simulink model "control_modos_deslizantes"  (R2016a)
settings: Solver=VariableStepAuto  StartTime=0.0  StopTime=20  RelTol=1e-3
undefined symbols (not defined in the file or in its folder): A, a0, a1, B, C, eta
settings Model: Creator=Daniel  LastModifiedBy=Daniel

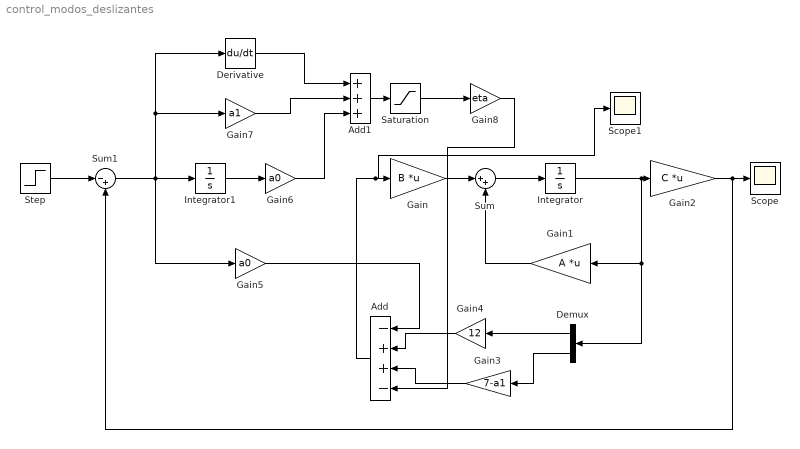
== system control_modos_deslizantes ==
  Add : Sum  Inputs=-++-
  Add1 : Sum  Inputs=+++
  Demux : Demux  Outputs=2
  Derivative : Derivative
  Gain : Gain  Gain=B  Multiplication=Matrix(K*u) (u vector)
  Gain1 : Gain  Gain=A  Multiplication=Matrix(K*u) (u vector)
  Gain2 : Gain  Gain=C  Multiplication=Matrix(K*u) (u vector)
  Gain3 : Gain  Gain=7-a1
  Gain4 : Gain  Gain=12
  Gain5 : Gain  Gain=a0
  Gain6 : Gain  Gain=a0
  Gain7 : Gain  Gain=a1
  Gain8 : Gain  Gain=eta
  Integrator : Integrator
  Integrator1 : Integrator
  Saturation : Saturate  UpperLimit=0.1  LowerLimit=-0.1
  Scope : Scope
  Scope1 : Scope
  Step : Step  SampleTime=0.1
  Sum : Sum  Inputs=|++
  Sum1 : Sum  Inputs=|-+
  wires:
  Sum/1 -> Integrator/1
  Gain1/1 -> Sum/2
  Gain/1 -> Sum/1
  Integrator/1 -> Demux/1, Gain1/1, Gain2/1
  Demux/1 -> Gain4/1
  Demux/2 -> Gain3/1
  Gain4/1 -> Add/2
  Gain3/1 -> Add/3
  Add/1 -> Scope1/1, Gain/1
  Gain2/1 -> Sum1/2, Scope/1
  Gain5/1 -> Add/1
  Sum1/1 -> Derivative/1, Gain7/1, Gain5/1, Integrator1/1
  Integrator1/1 -> Gain6/1
  Gain6/1 -> Add1/3
  Gain7/1 -> Add1/2
  Derivative/1 -> Add1/1
  Step/1 -> Sum1/1
  Add1/1 -> Saturation/1
  Saturation/1 -> Gain8/1
  Gain8/1 -> Add/4
